simulink model "PruebaSupervisoryLogic"  (R2022a)
settings: Solver=VariableStepAuto  StartTime=0.0  StopTime=100  RelTol=1e-3
values from neighbouring files (symbols this model uses):
  a = 0.2    [Data.m]
  alturaobst = 0.9    [Data.m]
  b = 0.542    [Data.m]
  M = [x_new y_new]    [Data.m]
  M_chasis = 3.5    [Data.m]
  M_rueda = 1    [Data.m]
  M_ruedacontacto = 1    [Data.m]
  N = 4365    [GraficasVelocidades.m]    (also in Prueba_Liapunov.m = length(p_X); WaypointsToTrayectory.m = length(X))
  R = 0.175/2    (= 0.0875)    [Data.m]
  X = M(:,1)    [WaypointsToTrayectory.m]
  x0 = x_ini(1)*factorE    [Data.m]
  x_obj = pos_fin(1)*factorE    [Data.m]
  xobstac = RandomPos(1)    [Data.m]
  Y = M(:, 2)    [WaypointsToTrayectory.m]
  y0 = y_ini(2)*factorE    [Data.m]
  y_obj = pos_fin(2)*factorE    [Data.m]
  yobstac = RandomPos(2)    [Data.m]
  zobstac = RandomPos(3)    [Data.m]
undefined symbols (not defined in the file or in its folder): bloqueobstaculo, Borde11, Borde12, Borde2, Borde3, Borde41, Borde42, Explanada, plano150g1, plano150g2, plano150g3, plano150g4, Plano150mm, plano150mm2irr, Plano45mm, plano45mm2irr, Plano90mm, Rampa, Rampa21, Rampa22, Rampa31, Rampa32, Rampa33, Rampa4, Rampa51, Rampa52, Rampa53, Terreno, Z
libraries: sm_lib x331, nesl_utility x30, fl_lib x3, robotalgslib x1
(part 8 of 8)

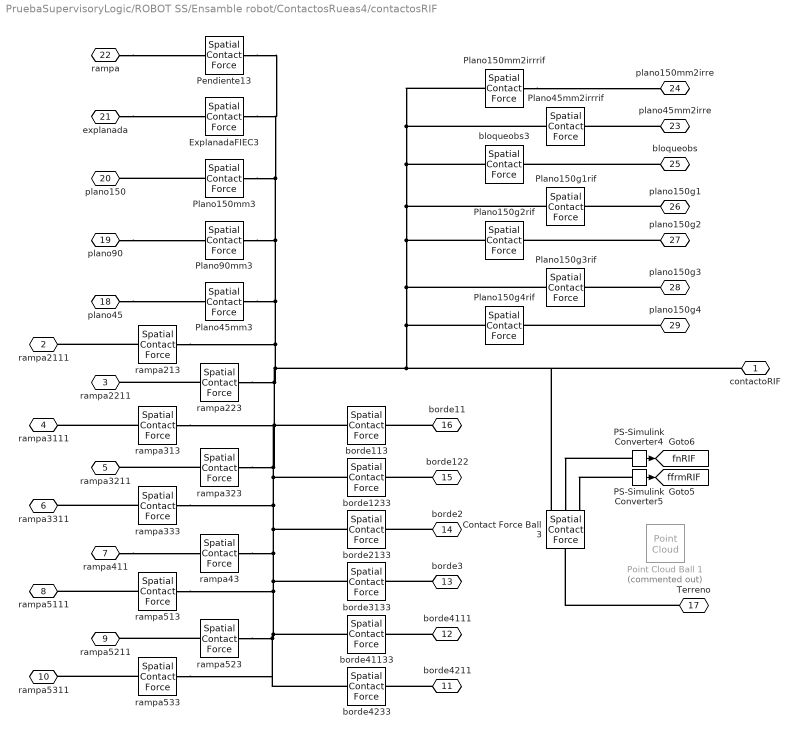
== system PruebaSupervisoryLogic/ROBOT SS/Ensamble robot/ContactosRueas4/contactosRIF ==
  Contact Force Ball 3 : sm_lib/Forces and Torques/Spatial Contact Force  SenseContactBaseRotation=off  SenseContactBaseTranslation=off  CoefficientOfDynamicFriction=0.5  CoefficientOfStaticFriction=0.8  NormalDamping=1000  NormalDampingUnits=N/(m/s)  SenseContactSignal=off  NormalStiffness=1000000  NormalStiffnessUnits=N/m  FrictionalCriticalVelocity=1e-3  FrictionalCriticalVelocityUnits=m/s  ZeroCrossDetectContactStartAndEnd=off  SenseContactFollowerRotation=off  SenseContactFollowerTranslation=off  FrictionType=SmoothStickSlip  SenseFrictionalForceMagnitude=on  SenseNormalForceMagnitude=on  NormalForceType=SmoothSpringDamper  SenseNormalVelocity=off  SenseSeparationDistance=off  SenseTangentialVelocity=off  NormalTransitionRegionWidth=1e-4  NormalTransitionRegionWidthUnits=m
  ExplanadaFIEC3 : sm_lib/Forces and Torques/Spatial Contact Force  SenseContactBaseRotation=off  SenseContactBaseTranslation=off  CoefficientOfDynamicFriction=0.3  CoefficientOfStaticFriction=0.5  NormalDamping=1e3  NormalDampingUnits=N/(m/s)  SenseContactSignal=off  NormalStiffness=1e6  NormalStiffnessUnits=N/m  FrictionalCriticalVelocity=1e-3  FrictionalCriticalVelocityUnits=m/s  ZeroCrossDetectContactStartAndEnd=off  SenseContactFollowerRotation=off  SenseContactFollowerTranslation=off  FrictionType=SmoothStickSlip  SenseFrictionalForceMagnitude=off  SenseNormalForceMagnitude=off  NormalForceType=SmoothSpringDamper  SenseNormalVelocity=off  SenseSeparationDistance=off  SenseTangentialVelocity=off  NormalTransitionRegionWidth=1e-4  NormalTransitionRegionWidthUnits=m
  PS-Simulink Converter4 : nesl_utility/PS-Simulink Converter  PhysicalDomain=network_engine_domain  SubClassName=ps_output  LeftPortType=input  RightPortType=output  PseudoPeriodic=off  Frequencies=[]  VectorFormat=inherit  Unit=inherit  AffineConversion=off
      settings: SourceProductBaseCode=SS,PW,VE
  PS-Simulink Converter5 : nesl_utility/PS-Simulink Converter  PhysicalDomain=network_engine_domain  SubClassName=ps_output  LeftPortType=input  RightPortType=output  PseudoPeriodic=off  Frequencies=[]  VectorFormat=inherit  Unit=inherit  AffineConversion=off
      settings: SourceProductBaseCode=SS,PW,VE
  Pendiente13 : sm_lib/Forces and Torques/Spatial Contact Force  SenseContactBaseRotation=off  SenseContactBaseTranslation=off  CoefficientOfDynamicFriction=0.3  CoefficientOfStaticFriction=0.5  NormalDamping=1e3  NormalDampingUnits=N/(m/s)  SenseContactSignal=off  NormalStiffness=1e6  NormalStiffnessUnits=N/m  FrictionalCriticalVelocity=1e-3  FrictionalCriticalVelocityUnits=m/s  ZeroCrossDetectContactStartAndEnd=off  SenseContactFollowerRotation=off  SenseContactFollowerTranslation=off  FrictionType=SmoothStickSlip  SenseFrictionalForceMagnitude=off  SenseNormalForceMagnitude=off  NormalForceType=SmoothSpringDamper  SenseNormalVelocity=off  SenseSeparationDistance=off  SenseTangentialVelocity=off  NormalTransitionRegionWidth=1e-4  NormalTransitionRegionWidthUnits=m
  Plano150g1rif : sm_lib/Forces and Torques/Spatial Contact Force  SenseContactBaseRotation=off  SenseContactBaseTranslation=off  CoefficientOfDynamicFriction=0.3  CoefficientOfStaticFriction=0.5  NormalDamping=1e3  NormalDampingUnits=N/(m/s)  SenseContactSignal=off  NormalStiffness=1e6  NormalStiffnessUnits=N/m  FrictionalCriticalVelocity=1e-3  FrictionalCriticalVelocityUnits=m/s  ZeroCrossDetectContactStartAndEnd=off  SenseContactFollowerRotation=off  SenseContactFollowerTranslation=off  FrictionType=SmoothStickSlip  SenseFrictionalForceMagnitude=off  SenseNormalForceMagnitude=off  NormalForceType=SmoothSpringDamper  SenseNormalVelocity=off  SenseSeparationDistance=off  SenseTangentialVelocity=off  NormalTransitionRegionWidth=1e-4  NormalTransitionRegionWidthUnits=m
  Plano150g2rif : sm_lib/Forces and Torques/Spatial Contact Force  SenseContactBaseRotation=off  SenseContactBaseTranslation=off  CoefficientOfDynamicFriction=0.3  CoefficientOfStaticFriction=0.5  NormalDamping=1e3  NormalDampingUnits=N/(m/s)  SenseContactSignal=off  NormalStiffness=1e6  NormalStiffnessUnits=N/m  FrictionalCriticalVelocity=1e-3  FrictionalCriticalVelocityUnits=m/s  ZeroCrossDetectContactStartAndEnd=off  SenseContactFollowerRotation=off  SenseContactFollowerTranslation=off  FrictionType=SmoothStickSlip  SenseFrictionalForceMagnitude=off  SenseNormalForceMagnitude=off  NormalForceType=SmoothSpringDamper  SenseNormalVelocity=off  SenseSeparationDistance=off  SenseTangentialVelocity=off  NormalTransitionRegionWidth=1e-4  NormalTransitionRegionWidthUnits=m
  Plano150g3rif : sm_lib/Forces and Torques/Spatial Contact Force  SenseContactBaseRotation=off  SenseContactBaseTranslation=off  CoefficientOfDynamicFriction=0.3  CoefficientOfStaticFriction=0.5  NormalDamping=1e3  NormalDampingUnits=N/(m/s)  SenseContactSignal=off  NormalStiffness=1e6  NormalStiffnessUnits=N/m  FrictionalCriticalVelocity=1e-3  FrictionalCriticalVelocityUnits=m/s  ZeroCrossDetectContactStartAndEnd=off  SenseContactFollowerRotation=off  SenseContactFollowerTranslation=off  FrictionType=SmoothStickSlip  SenseFrictionalForceMagnitude=off  SenseNormalForceMagnitude=off  NormalForceType=SmoothSpringDamper  SenseNormalVelocity=off  SenseSeparationDistance=off  SenseTangentialVelocity=off  NormalTransitionRegionWidth=1e-4  NormalTransitionRegionWidthUnits=m
  Plano150g4rif : sm_lib/Forces and Torques/Spatial Contact Force  SenseContactBaseRotation=off  SenseContactBaseTranslation=off  CoefficientOfDynamicFriction=0.3  CoefficientOfStaticFriction=0.5  NormalDamping=1e3  NormalDampingUnits=N/(m/s)  SenseContactSignal=off  NormalStiffness=1e6  NormalStiffnessUnits=N/m  FrictionalCriticalVelocity=1e-3  FrictionalCriticalVelocityUnits=m/s  ZeroCrossDetectContactStartAndEnd=off  SenseContactFollowerRotation=off  SenseContactFollowerTranslation=off  FrictionType=SmoothStickSlip  SenseFrictionalForceMagnitude=off  SenseNormalForceMagnitude=off  NormalForceType=SmoothSpringDamper  SenseNormalVelocity=off  SenseSeparationDistance=off  SenseTangentialVelocity=off  NormalTransitionRegionWidth=1e-4  NormalTransitionRegionWidthUnits=m
  Plano150mm2irrrif : sm_lib/Forces and Torques/Spatial Contact Force  SenseContactBaseRotation=off  SenseContactBaseTranslation=off  CoefficientOfDynamicFriction=0.3  CoefficientOfStaticFriction=0.5  NormalDamping=1e3  NormalDampingUnits=N/(m/s)  SenseContactSignal=off  NormalStiffness=1e6  NormalStiffnessUnits=N/m  FrictionalCriticalVelocity=1e-3  FrictionalCriticalVelocityUnits=m/s  ZeroCrossDetectContactStartAndEnd=off  SenseContactFollowerRotation=off  SenseContactFollowerTranslation=off  FrictionType=SmoothStickSlip  SenseFrictionalForceMagnitude=off  SenseNormalForceMagnitude=off  NormalForceType=SmoothSpringDamper  SenseNormalVelocity=off  SenseSeparationDistance=off  SenseTangentialVelocity=off  NormalTransitionRegionWidth=1e-4  NormalTransitionRegionWidthUnits=m
  Plano150mm3 : sm_lib/Forces and Torques/Spatial Contact Force  SenseContactBaseRotation=off  SenseContactBaseTranslation=off  CoefficientOfDynamicFriction=0.3  CoefficientOfStaticFriction=0.5  NormalDamping=1e3  NormalDampingUnits=N/(m/s)  SenseContactSignal=off  NormalStiffness=1e6  NormalStiffnessUnits=N/m  FrictionalCriticalVelocity=1e-3  FrictionalCriticalVelocityUnits=m/s  ZeroCrossDetectContactStartAndEnd=off  SenseContactFollowerRotation=off  SenseContactFollowerTranslation=off  FrictionType=SmoothStickSlip  SenseFrictionalForceMagnitude=off  SenseNormalForceMagnitude=off  NormalForceType=SmoothSpringDamper  SenseNormalVelocity=off  SenseSeparationDistance=off  SenseTangentialVelocity=off  NormalTransitionRegionWidth=1e-4  NormalTransitionRegionWidthUnits=m
  Plano45mm2irrrif : sm_lib/Forces and Torques/Spatial Contact Force  SenseContactBaseRotation=off  SenseContactBaseTranslation=off  CoefficientOfDynamicFriction=0.3  CoefficientOfStaticFriction=0.5  NormalDamping=1e3  NormalDampingUnits=N/(m/s)  SenseContactSignal=off  NormalStiffness=1e6  NormalStiffnessUnits=N/m  FrictionalCriticalVelocity=1e-3  FrictionalCriticalVelocityUnits=m/s  ZeroCrossDetectContactStartAndEnd=off  SenseContactFollowerRotation=off  SenseContactFollowerTranslation=off  FrictionType=SmoothStickSlip  SenseFrictionalForceMagnitude=off  SenseNormalForceMagnitude=off  NormalForceType=SmoothSpringDamper  SenseNormalVelocity=off  SenseSeparationDistance=off  SenseTangentialVelocity=off  NormalTransitionRegionWidth=1e-4  NormalTransitionRegionWidthUnits=m
  Plano45mm3 : sm_lib/Forces and Torques/Spatial Contact Force  SenseContactBaseRotation=off  SenseContactBaseTranslation=off  CoefficientOfDynamicFriction=0.3  CoefficientOfStaticFriction=0.5  NormalDamping=1e3  NormalDampingUnits=N/(m/s)  SenseContactSignal=off  NormalStiffness=1e6  NormalStiffnessUnits=N/m  FrictionalCriticalVelocity=1e-3  FrictionalCriticalVelocityUnits=m/s  ZeroCrossDetectContactStartAndEnd=off  SenseContactFollowerRotation=off  SenseContactFollowerTranslation=off  FrictionType=SmoothStickSlip  SenseFrictionalForceMagnitude=off  SenseNormalForceMagnitude=off  NormalForceType=SmoothSpringDamper  SenseNormalVelocity=off  SenseSeparationDistance=off  SenseTangentialVelocity=off  NormalTransitionRegionWidth=1e-4  NormalTransitionRegionWidthUnits=m
  Plano90mm3 : sm_lib/Forces and Torques/Spatial Contact Force  SenseContactBaseRotation=off  SenseContactBaseTranslation=off  CoefficientOfDynamicFriction=0.3  CoefficientOfStaticFriction=0.5  NormalDamping=1e3  NormalDampingUnits=N/(m/s)  SenseContactSignal=off  NormalStiffness=1e6  NormalStiffnessUnits=N/m  FrictionalCriticalVelocity=1e-3  FrictionalCriticalVelocityUnits=m/s  ZeroCrossDetectContactStartAndEnd=off  SenseContactFollowerRotation=off  SenseContactFollowerTranslation=off  FrictionType=SmoothStickSlip  SenseFrictionalForceMagnitude=off  SenseNormalForceMagnitude=off  NormalForceType=SmoothSpringDamper  SenseNormalVelocity=off  SenseSeparationDistance=off  SenseTangentialVelocity=off  NormalTransitionRegionWidth=1e-4  NormalTransitionRegionWidthUnits=m
  Point Cloud Ball 1 : sm_lib/Curves and Surfaces/Point Cloud  Commented=on  CoordinatesMatrix=rueda_ptcld  CoordinatesMatrixUnits=m  GraphicType=MarkerCloud  GraphicSphereRadius=0.001  GraphicSphereRadiusUnits=m  GraphicVisPropType=SimpleVisualProperties  GraphicDiffuseColor=[1 0 0]  GraphicOpacity=1  GraphicSpecularColor=[0.5 0.5 0.5 1.0]  GraphicAmbientColor=[0.15 0.15 0.15 1.0]  GraphicEmissiveColor=[0.0 0.0 0.0 1.0]  GraphicShininess=75
      settings: SourceProductBaseCode=MS
  bloqueobs3 : sm_lib/Forces and Torques/Spatial Contact Force  SenseContactBaseRotation=off  SenseContactBaseTranslation=off  CoefficientOfDynamicFriction=0.3  CoefficientOfStaticFriction=0.5  NormalDamping=1e3  NormalDampingUnits=N/(m/s)  SenseContactSignal=off  NormalStiffness=1e6  NormalStiffnessUnits=N/m  FrictionalCriticalVelocity=1e-3  FrictionalCriticalVelocityUnits=m/s  ZeroCrossDetectContactStartAndEnd=off  SenseContactFollowerRotation=off  SenseContactFollowerTranslation=off  FrictionType=SmoothStickSlip  SenseFrictionalForceMagnitude=off  SenseNormalForceMagnitude=off  NormalForceType=SmoothSpringDamper  SenseNormalVelocity=off  SenseSeparationDistance=off  SenseTangentialVelocity=off  NormalTransitionRegionWidth=1e-4  NormalTransitionRegionWidthUnits=m
  borde{113,1233,2133,3133,4233,41133} (6 alike) : sm_lib/Forces and Torques/Spatial Contact Force  SenseContactBaseRotation=off  SenseContactBaseTranslation=off  CoefficientOfDynamicFriction=0.3  CoefficientOfStaticFriction=0.5  NormalDamping=1e3  NormalDampingUnits=N/(m/s)  SenseContactSignal=off  NormalStiffness=1e6  NormalStiffnessUnits=N/m  FrictionalCriticalVelocity=1e-3  FrictionalCriticalVelocityUnits=m/s  ZeroCrossDetectContactStartAndEnd=off  SenseContactFollowerRotation=off  SenseContactFollowerTranslation=off  FrictionType=SmoothStickSlip  SenseFrictionalForceMagnitude=off  SenseNormalForceMagnitude=off  NormalForceType=SmoothSpringDamper  SenseNormalVelocity=off  SenseSeparationDistance=off  SenseTangentialVelocity=off  NormalTransitionRegionWidth=1e-4  NormalTransitionRegionWidthUnits=m
  rampa{43,213,223,313,323,333,513,523,533} (9 alike) : sm_lib/Forces and Torques/Spatial Contact Force  SenseContactBaseRotation=off  SenseContactBaseTranslation=off  CoefficientOfDynamicFriction=0.3  CoefficientOfStaticFriction=0.5  NormalDamping=1e3  NormalDampingUnits=N/(m/s)  SenseContactSignal=off  NormalStiffness=1e6  NormalStiffnessUnits=N/m  FrictionalCriticalVelocity=1e-3  FrictionalCriticalVelocityUnits=m/s  ZeroCrossDetectContactStartAndEnd=off  SenseContactFollowerRotation=off  SenseContactFollowerTranslation=off  FrictionType=SmoothStickSlip  SenseFrictionalForceMagnitude=off  SenseNormalForceMagnitude=off  NormalForceType=SmoothSpringDamper  SenseNormalVelocity=off  SenseSeparationDistance=off  SenseTangentialVelocity=off  NormalTransitionRegionWidth=1e-4  NormalTransitionRegionWidthUnits=m
  contactoRIF : PMIOPort  Side=Left
  rampa2111 : PMIOPort  Port=2  Side=Left
  rampa2211 : PMIOPort  Port=3  Side=Left
  rampa3111 : PMIOPort  Port=4  Side=Left
  rampa3211 : PMIOPort  Port=5  Side=Left
  rampa3311 : PMIOPort  Port=6  Side=Left
  rampa411 : PMIOPort  Port=7  Side=Left
  rampa5111 : PMIOPort  Port=8  Side=Left
  rampa5211 : PMIOPort  Port=9  Side=Left
  rampa5311 : PMIOPort  Port=10  Side=Left
  borde4211 : PMIOPort  Port=11  Side=Right
  borde4111 : PMIOPort  Port=12  Side=Right
  borde3 : PMIOPort  Port=13  Side=Right
  borde2 : PMIOPort  Port=14  Side=Right
  borde122 : PMIOPort  Port=15  Side=Right
  borde11 : PMIOPort  Port=16  Side=Right
  Terreno : PMIOPort  Port=17  Side=Right
  plano45 : PMIOPort  Port=18  Side=Right
  plano90 : PMIOPort  Port=19  Side=Right
  plano150 : PMIOPort  Port=20  Side=Right
  explanada : PMIOPort  Port=21  Side=Right
  rampa : PMIOPort  Port=22  Side=Right
  plano45mm2irre : PMIOPort  Port=23  Side=Right
  plano150mm2irre : PMIOPort  Port=24  Side=Right
  bloqueobs : PMIOPort  Port=25  Side=Right
  plano150g1 : PMIOPort  Port=26  Side=Right
  plano150g2 : PMIOPort  Port=27  Side=Right
  plano150g3 : PMIOPort  Port=28  Side=Right
  plano150g4 : PMIOPort  Port=29  Side=Right
  tag scope: ffrmRIF=global, fnRIF=global
  wires:
  PS-Simulink Converter5/1 -> [ffrmRIF]
  PS-Simulink Converter4/1 -> [fnRIF]
  connections:
  Plano150mm2irrrif/RConn1 -- bloqueobs3/RConn1 -- Plano150g1rif/RConn1 -- Plano150g2rif/RConn1 -- Plano150g3rif/RConn1 -- Plano150g4rif/RConn1 -- rampa213/RConn1 -- Plano90mm3/RConn1 -- Pendiente13/RConn1 -- ExplanadaFIEC3/RConn1 -- Plano150mm3/RConn1 -- Plano45mm3/RConn1 -- rampa333/RConn1 -- borde2133/LConn1 -- borde3133/LConn1 -- borde41133/LConn1 -- borde4233/LConn1 -- rampa533/RConn1 -- rampa523/RConn1 -- rampa513/RConn1 -- rampa43/RConn1 -- borde1233/LConn1 -- rampa323/RConn1 -- borde113/LConn1 -- rampa313/RConn1 -- rampa223/RConn1 -- Contact Force Ball 3/RConn1 -- contactoRIF/RConn1 -- Plano45mm2irrrif/RConn1
  Plano150mm3/LConn1 -- plano150/RConn1
  plano90/RConn1 -- Plano90mm3/LConn1
  plano45/RConn1 -- Plano45mm3/LConn1
  rampa/RConn1 -- Pendiente13/LConn1
  PS-Simulink Converter4/LConn1 -- Contact Force Ball 3/RConn2
  explanada/RConn1 -- ExplanadaFIEC3/LConn1
  Terreno/RConn1 -- Contact Force Ball 3/LConn1
  PS-Simulink Converter5/LConn1 -- Contact Force Ball 3/RConn3
  rampa213/LConn1 -- rampa2111/RConn1
  rampa333/LConn1 -- rampa3311/RConn1
  rampa513/LConn1 -- rampa5111/RConn1
  rampa533/LConn1 -- rampa5311/RConn1
  rampa523/LConn1 -- rampa5211/RConn1
  rampa223/LConn1 -- rampa2211/RConn1
  rampa313/LConn1 -- rampa3111/RConn1
  rampa411/RConn1 -- rampa43/LConn1
  rampa323/LConn1 -- rampa3211/RConn1
  borde4211/RConn1 -- borde4233/RConn1
  borde122/RConn1 -- borde1233/RConn1
  borde3/RConn1 -- borde3133/RConn1
  borde11/RConn1 -- borde113/RConn1
  borde4111/RConn1 -- borde41133/RConn1
  borde2/RConn1 -- borde2133/RConn1
  plano150g4/RConn1 -- Plano150g4rif/LConn1
  bloqueobs/RConn1 -- bloqueobs3/LConn1
  plano150g2/RConn1 -- Plano150g2rif/LConn1
  plano150g1/RConn1 -- Plano150g1rif/LConn1
  plano150g3/RConn1 -- Plano150g3rif/LConn1
  Plano150mm2irrrif/LConn1 -- plano150mm2irre/RConn1
  plano45mm2irre/RConn1 -- Plano45mm2irrrif/LConn1

== system PruebaSupervisoryLogic/ROBOT SS/Ensamble robot/Tapa/Frontal ==
  Cylindrical Solid : sm_lib/Body Elements/Cylindrical Solid  GraphicAmbientColor=[0.15 0.15 0.15 1.0]  BasedOnType=Density  CenterOfMass=[0 0 0]  CenterOfMassUnits=m  GraphicDiffuseColor=[0.5 0.5 0.5]  CylinderLength=0.3  CylinderLengthUnits=m  CylinderRadius=0.1  CylinderRadiusUnits=m  Density=1000  DensityUnits=kg/m^3  DoExposeReferenceFrame=on  GraphicEmissiveColor=[0.0 0.0 0.0 1.0]  ExportEntireGeometry=off  SerializedFrames=<Frames><Frame><Id>Frame1</Id><Value><Name>F1</Name><Origin><Source>GeometricFeature</Source><FeatureName>top curve</FeatureName></Origin><PrimaryAxis><DefinedDirection>+X</DefinedDirection><Source>GeometricFeature</Source><SourceDirection>+Z</SourceDirection><FeatureName>top curve</FeatureName></PrimaryAxis><SecondaryAxis><DefinedDirection>-Z</DefinedDirection><Source>ReferenceFrame</Source><SourceDirection>+X</SourceDirection><FeatureName></FeatureName></SecondaryAxis></Value></Frame></Frames>  MarkerShape=Sphere  MarkerSize=10  GraphicType=None  InertiaType=CalculateFromGeometry  Mass=1  MassUnits=kg  MomentsOfInertia=[1 1 1]  MomentsOfInertiaUnits=kg*m^2  GraphicOpacity=1.0  ProductsOfInertia=[0 0 0]  ProductsOfInertiaUnits=kg*m^2  GraphicShininess=75  GraphicSpecularColor=[0.5 0.5 0.5 1.0]  GraphicVisPropType=SimpleVisualProperties
  Cylindrical Solid1 : sm_lib/Body Elements/Cylindrical Solid  GraphicAmbientColor=[0.15 0.15 0.15 1.0]  BasedOnType=Density  CenterOfMass=[0 0 0]  CenterOfMassUnits=m  GraphicDiffuseColor=[0.5 0.5 0.5]  CylinderLength=0.1  CylinderLengthUnits=m  CylinderRadius=0.1  CylinderRadiusUnits=m  Density=1000  DensityUnits=kg/m^3  DoExposeReferenceFrame=on  GraphicEmissiveColor=[0.0 0.0 0.0 1.0]  ExportEntireGeometry=off  SerializedFrames=<Frames/>  MarkerShape=Sphere  MarkerSize=10  GraphicType=None  InertiaType=CalculateFromGeometry  Mass=1  MassUnits=kg  MomentsOfInertia=[1 1 1]  MomentsOfInertiaUnits=kg*m^2  GraphicOpacity=1.0  ProductsOfInertia=[0 0 0]  ProductsOfInertiaUnits=kg*m^2  GraphicShininess=75  GraphicSpecularColor=[0.5 0.5 0.5 1.0]  GraphicVisPropType=SimpleVisualProperties
  Conn1 : PMIOPort  Side=Right
  connections:
  Cylindrical Solid1/RConn1 -- Cylindrical Solid/LConn1
  Cylindrical Solid/RConn1 -- Conn1/RConn1

== matlab function PruebaSupervisoryLogic/ROBOT SS/DOF/theta_act ==
  data: u input; z output; y output; x output
function [z,y,x] = fcn(u)
out = quat2eul(u');
z = out(1);
y = out(2);
x = out(3);
end

== matlab function PruebaSupervisoryLogic/Sensores Frente x7/Percepción_Central/SensorUltrasonido2/MATLAB Function ==
  data: Obs_Pose input; d output; PhiSensor input; R_Pose input; di_sensor input; d_real output
function [d, d_real]= fcn(Obs_Pose, PhiSensor, R_Pose, di_sensor)

x_Robot = R_Pose(1);
y_Robot = R_Pose(2);
tetha_Robot = R_Pose(3);

x_Obst= Obs_Pose(1);
y_Obst= Obs_Pose(2);


%Calcular la distancia entre la pose del robot 
distance = sqrt((x_Robot - x_Obst)^2 + (y_Robot - y_Obst)^2);
d_real= distance-di_sensor;

%Calcular angulo
betha = atan(abs((y_Obst - y_Robot)/(x_Obst- x_Robot)));

fi = betha-tetha_Robot;

if (abs(fi-PhiSensor) <= 0.1)


    d = d_real;
 
else
    d= 1000;
end

== stateflow chart PruebaSupervisoryLogic/Path Planning1/Waypoint Tracking Logic ==
  state FollowWaypoints
    entry:
    goalPoint = waypoints(idx,:);
    entry, during:
    [angle,range] = trackGoal(goalPoint);
    (default) -> (junction 20)
    FollowWaypoints -> (junction 20) [order 1]
    (junction 20) -> (junction 24) [order 1] : % Set angular speed if
        | % angle outside deadband
        | [abs(angle) > pi/24]
    (junction 20) -> (junction 30) [order 2] : {w = 0;}
    (junction 24) -> (junction 49) : % Proportional
        | % control
        | {w = 20*angle}
    (junction 49) -> (junction 30)
  state ReachedGoal
    entry:
    v = 0;
    w = 0.5;
  (default) -> FollowWaypoints : {
      | v = 1.38;
      | idx = 1;
      | numPts = size(waypoints,1);
      | }
  FollowWaypoints -> (junction 39) [order 1] : % Check if goal reached
      | [range < 0.1]
  (junction 39) -> ReachedGoal [order 1] : % Stop if final waypoint
      | [idx == numPts]
  (junction 39) -> (junction 42) [order 2]
  (junction 42) -> FollowWaypoints : % Go to the next waypoint
      | {idx = idx + 1;}
  data: goal function_input; ang function_output; dist function_output; pose input; waypoints input; v output; w output; angle local; range local; idx local; numPts local; goalPoint local
  function [ang,dist] = trackGoal(goal):
    | function [ang,dist] = trackGoal(goal)
    | % Finds the angle (theta) and distance (dist) between the 
    | % vehicle and a goal point
    |     
    | posDiff = [goal(1)-pose(1);goal(2)-pose(2)];
    | 
    | ang = angdiff(pose(3),atan2(posDiff(2),posDiff(1)));
    | dist = sqrt(posDiff(1)^2 + posDiff(2)^2);

== matlab function PruebaSupervisoryLogic/Sensores Frente x7/Percepción_Izquierda/SensorUltrasonido/MATLAB Function ==
  data: Obs_Pose input; d output; PhiSensor input; R_Pose input; di_sensor input; d_real output
function [d, d_real]= fcn(Obs_Pose, PhiSensor, R_Pose, di_sensor)

x_Robot = R_Pose(1);
y_Robot = R_Pose(2);
tetha_Robot = R_Pose(3);

x_Obst= Obs_Pose(1);
y_Obst= Obs_Pose(2);


%Calcular la distancia entre la pose del robot 
distance = sqrt((x_Robot - x_Obst)^2 + (y_Robot - y_Obst)^2);
d_real= distance-di_sensor;

%Calcular angulo
betha = atan(abs((y_Obst - y_Robot)/(x_Obst- x_Robot)));

fi = betha-tetha_Robot;

if (abs(fi-PhiSensor) <= 0.1)


    d = d_real;
 
else
    d= 1000;
end

== matlab function PruebaSupervisoryLogic/Sensores Frente x7/Percepción_Izquierda/SensorUltrasonido1/MATLAB Function ==
  data: Obs_Pose input; d output; PhiSensor input; R_Pose input; di_sensor input; d_real output
function [d, d_real]= fcn(Obs_Pose, PhiSensor, R_Pose, di_sensor)

x_Robot = R_Pose(1);
y_Robot = R_Pose(2);
tetha_Robot = R_Pose(3);

x_Obst= Obs_Pose(1);
y_Obst= Obs_Pose(2);


%Calcular la distancia entre la pose del robot 
distance = sqrt((x_Robot - x_Obst)^2 + (y_Robot - y_Obst)^2);
d_real= distance-di_sensor;

%Calcular angulo
betha = atan(abs((y_Obst - y_Robot)/(x_Obst- x_Robot)));

fi = betha-tetha_Robot;

if (abs(fi-PhiSensor) <= 0.1)


    d = d_real;
 
else
    d= 1000;
end

== matlab function PruebaSupervisoryLogic/Sensores Frente x7/Percepción_Derecha/SensorUltrasonido/MATLAB Function ==
  data: Obs_Pose input; d output; PhiSensor input; R_Pose input; di_sensor input; d_real output
function [d, d_real]= fcn(Obs_Pose, PhiSensor, R_Pose, di_sensor)

x_Robot = R_Pose(1);
y_Robot = R_Pose(2);
tetha_Robot = R_Pose(3);

x_Obst= Obs_Pose(1);
y_Obst= Obs_Pose(2);


%Calcular la distancia entre la pose del robot 
distance = sqrt((x_Robot - x_Obst)^2 + (y_Robot - y_Obst)^2);
d_real= distance-di_sensor;

%Calcular angulo
betha = atan(abs((y_Obst - y_Robot)/(x_Obst- x_Robot)));

fi = betha-tetha_Robot;

if (abs(fi-PhiSensor) <= 0.1)


    d = d_real;
 
else
    d= 1000;
end

== matlab function PruebaSupervisoryLogic/Sensores Frente x7/Percepción_Derecha/SensorUltrasonido1/MATLAB Function ==
  data: Obs_Pose input; d output; PhiSensor input; R_Pose input; di_sensor input; d_real output
function [d, d_real]= fcn(Obs_Pose, PhiSensor, R_Pose, di_sensor)

x_Robot = R_Pose(1);
y_Robot = R_Pose(2);
tetha_Robot = R_Pose(3);

x_Obst= Obs_Pose(1);
y_Obst= Obs_Pose(2);


%Calcular la distancia entre la pose del robot 
distance = sqrt((x_Robot - x_Obst)^2 + (y_Robot - y_Obst)^2);
d_real= distance-di_sensor;

%Calcular angulo
betha = atan(abs((y_Obst - y_Robot)/(x_Obst- x_Robot)));

fi = betha-tetha_Robot;

if (abs(fi-PhiSensor) <= 0.1)


    d = d_real;
 
else
    d= 1000;
end

== matlab function PruebaSupervisoryLogic/Path Planning2/Kinematics1/Direct-Kinematics/MATLAB Function ==
  data: xp output; yp output; wr input; wl input; r input; c input; a input; o output; or input
function [xp,yp,o] = fcn(wr,wl,r,c,a, or)

o= or;

v1= c*cos(o) - 2*a*sin(o);
v2= c*cos(o) + 2*a*sin(o);
v3= c*sin(o) + 2*a*cos(o);
v4= c*sin(o) - 2*a*cos(o);

xp=(r/(2*c))*(v1*wr+v2*wl);
yp= (r/(2*c))*(v3*wr+v4*wl);

== matlab function PruebaSupervisoryLogic/Path Planning2/Subsystem1/check-goal/MATLAB Function ==
  data: posexy input; distanceGoal output; goal input
function distanceGoal  = fcn( posexy, goal)

distanceGoal = sqrt(((goal(1)-posexy(1))^2)+ ((goal(2)-posexy(2))^2) );
end

== matlab function PruebaSupervisoryLogic/Path Planning2/Trapezoidal Vel Profile ==
  data: linVel input; t input; t1 input; lin_Vel_out output; accel input; deaccelStartTime input
function lin_Vel_out = fcn(linVel,t,t1,accel,deaccelStartTime)
% Function to create a trapezoidal profile for rover's desired linear
% velocity

t2 = linVel/accel + t1;
t3 = deaccelStartTime + 0.2;
tf = linVel/accel + t3;

if t>=t1 && t<t2 
    lin_Vel_out = accel*(t-t1);

elseif t>=t2 && t < t3 
    lin_Vel_out = linVel;

elseif t>= t3 && t < tf 
    lin_Vel_out = linVel-accel*(t-t3);

else
    lin_Vel_out = 0;    
end


end

== matlab function PruebaSupervisoryLogic/ROBOT SS/Promedio ==
  data: wr output; wl output; w1 input; w2 input; w3 input; w4 input
function [wr, wl] = Promedio(w1,w2,w3,w4)

wr= (w1+w2)/(2);
wl= (w3+w4)/(2);

== matlab function PruebaSupervisoryLogic/ROBOT SS/Subsystem/Rot 2 eul ==
  data: z output; R input
function z  = fcn(R)
out = rotm2eul(R);
z = out(1);
end

== matlab function PruebaSupervisoryLogic/ROBOT SS/Subsystem/Vlineal ==
  data: vx input; v output; vy input
function v = fcn(vx, vy)

v = sqrt((vx)^2 + (vy)^2);
end

== matlab function PruebaSupervisoryLogic/Sensores Frente x7/Percepción_Central/SensorUltrasonido/MATLAB Function ==
  data: Obs_Pose input; d output; PhiSensor input; R_Pose input; di_sensor input; d_real output
function [d, d_real]= fcn(Obs_Pose, PhiSensor, R_Pose, di_sensor)

x_Robot = R_Pose(1);
y_Robot = R_Pose(2);
tetha_Robot = R_Pose(3);

x_Obst= Obs_Pose(1);
y_Obst= Obs_Pose(2);


%Calcular la distancia entre la pose del robot 
distance = sqrt((x_Robot - x_Obst)^2 + (y_Robot - y_Obst)^2);
d_real= distance-di_sensor;

%Calcular angulo
betha = atan(abs((y_Obst - y_Robot)/(x_Obst- x_Robot)));

fi = betha-tetha_Robot;

if (abs(fi-PhiSensor) <= 0.1)


    d = d_real;
 
else
    d= 1000;
end

== matlab function PruebaSupervisoryLogic/Sensores Frente x7/Percepción_Central/SensorUltrasonido1/MATLAB Function ==
  data: Obs_Pose input; d output; PhiSensor input; R_Pose input; di_sensor input; d_real output
function [d, d_real]= fcn(Obs_Pose, PhiSensor, R_Pose, di_sensor)

x_Robot = R_Pose(1);
y_Robot = R_Pose(2);
tetha_Robot = R_Pose(3);

x_Obst= Obs_Pose(1);
y_Obst= Obs_Pose(2);


%Calcular la distancia entre la pose del robot 
distance = sqrt((x_Robot - x_Obst)^2 + (y_Robot - y_Obst)^2);
d_real= distance-di_sensor;

%Calcular angulo
betha = atan(abs((y_Obst - y_Robot)/(x_Obst- x_Robot)));

fi = betha-tetha_Robot;

if (abs(fi-PhiSensor) <= 0.1)


    d = d_real;
 
else
    d= 1000;
end
